simulink model "VTOL_sim_8_f_Mk2"  (R2018a)
settings: Solver=VariableStepAuto  StartTime=0.0  StopTime=20  RelTol=1e-3
InitFcn:
  | vtol_param
StartFcn:
  | vtol_param
undefined symbols (not defined in the file or in its folder): P, PlotVtol
ContinueFcn:
  | FT2frfl
settings Model: Creator=sadam  LastModifiedBy=sadam

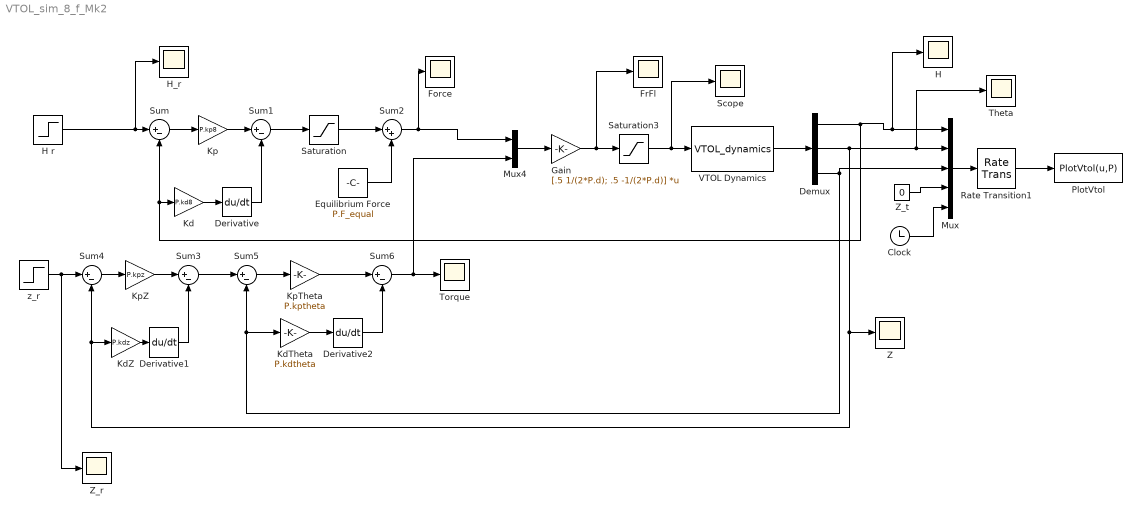
== system VTOL_sim_8_f_Mk2 ==
  Clock : Clock
  Demux : Demux  Outputs=3
  Derivative : Derivative
  Derivative1 : Derivative
  Derivative2 : Derivative
  Equilibrium Force : Constant  Value=P.F_equal
  Force : Scope
  FrFl : Scope
  Gain : Gain  Gain=[.5 1/(2*P.d); .5 -1/(2*P.d)]  Multiplication=Matrix(K*u)
  H : Scope
  H r : Step  After=3  SampleTime=0
  H_r : Scope
  Kd : Gain  Gain=P.kd8
  "KdTheta " : Gain  Gain=P.kdtheta
  "KdZ " : Gain  Gain=P.kdz
  Kp : Gain  Gain=P.kp8
  "KpTheta " : Gain  Gain=P.kptheta
  "KpZ " : Gain  Gain=P.kpz
  Mux : Mux  Inputs=5
  Mux4 : Mux  Inputs=2
  "PlotVtol " : MATLABFcn  MATLABFcn=PlotVtol(u,P)  OutputDimensions=0
  Rate Transition1 : RateTransition  OutPortSampleTime=P.t_plot
  Saturation : Saturate  UpperLimit=P.Force_max  LowerLimit=-P.Force_max
  Saturation3 : Saturate  UpperLimit=P.Force_max  LowerLimit=-P.Force_max
  Scope : Scope
  Sum{,1,3..6} (6 alike) : Sum  Inputs=|+-
  Sum2 : Sum  Inputs=|++
  "Theta " : Scope
  Torque : Scope
  VTOL Dynamics : S-Function  FunctionName=VTOL_dynamics  Parameters=P  SFunctionDeploymentMode=off  EnableBusSupport=off
  Z : Scope
  "Z_r " : Scope
  Z_t : Constant  Value=0
  "z_r " : Step  After=3  SampleTime=0
  wires:
  Sum/1 -> Kp/1
  Kd/1 -> Derivative/1
  Kp/1 -> Sum1/1
  Derivative/1 -> Sum1/2
  Mux/1 -> Rate Transition1/1
  VTOL Dynamics/1 -> Demux/1
  Saturation/1 -> Sum2/1
  Equilibrium Force/1 -> Sum2/2
  Sum1/1 -> Saturation/1
  Rate Transition1/1 -> "PlotVtol "/1
  Z_t/1 -> Mux/4
  Clock/1 -> Mux/5
  "KpZ "/1 -> Sum3/1
  Sum4/1 -> "KpZ "/1
  Sum3/1 -> Sum5/1
  "KdZ "/1 -> Derivative1/1
  Derivative1/1 -> Sum3/2
  Sum5/1 -> "KpTheta "/1
  "KdTheta "/1 -> Derivative2/1
  "KpTheta "/1 -> Sum6/1
  Derivative2/1 -> Sum6/2
  Demux/1 -> H/1, Mux/1, Kd/1, Sum/2
  Sum2/1 -> Force/1, Mux4/1
  Sum6/1 -> Mux4/2, Torque/1
  H r/1 -> H_r/1, Sum/1
  Demux/2 -> Z/1, "KdZ "/1, Sum4/2, "Theta "/1, Mux/2
  Demux/3 -> Mux/3, "KdTheta "/1, Sum5/2
  "z_r "/1 -> "Z_r "/1, Sum4/1
  Saturation3/1 -> Scope/1, VTOL Dynamics/1
  Gain/1 -> FrFl/1, Saturation3/1
  Mux4/1 -> Gain/1
